simulink model "Probleme25"  (R2024a)
settings: Solver=VariableStepAuto  StartTime=0.0  StopTime=100.0  RelTol=1e-3
settings Model: Creator=francoisdesautels  LastModifiedBy=francoisdesautels

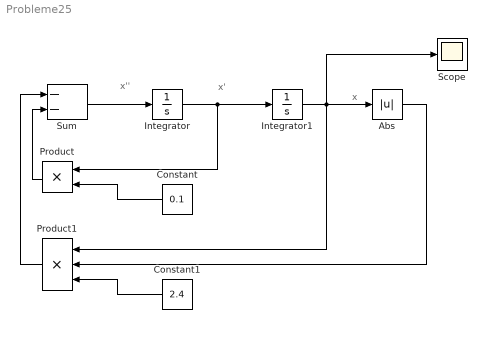
== system Probleme25 ==
  note: x
  note: x'
  note: x''
  Abs : Abs  SaturateOnIntegerOverflow=off
  Constant : Constant  Value=0.1
  Constant1 : Constant  Value=2.4
  Integrator : Integrator  InitialCondition=0.2
  Integrator1 : Integrator  InitialCondition=0.2
  Product : Product
  Product1 : Product  Inputs=3
  Scope : Scope
  Sum : Sum  Inputs=--
  wires:
  Product/1 -> Sum/2
  Integrator/1 -> Integrator1/1, Product/1
  Constant/1 -> Product/2
  Sum/1 -> Integrator/1
  Integrator1/1 -> Scope/1, Abs/1, Product1/1
  Abs/1 -> Product1/2
  Constant1/1 -> Product1/3
  Product1/1 -> Sum/1
